simulink model "uas_sim"  (R2023a)
settings: Solver=VariableStepAuto  StartTime=0.0  StopTime=10.0  RelTol=1e-3  SampleTimeConstraint=STIndependent
values from neighbouring files (symbols this model uses):
  framePeriod_s = 1/frameRate_hz    (= 0.02)    [setup.m]
undefined symbols (not defined in the file or in its folder): Aircraft, datetime, datevec, Earth, Env, Fmu, InitCond, Telem, WGS84
libraries: aerolibconvert2 x8, simulink x8, aerolibadyn x3, aerolibasang x3, aerolibtransform2 x2, aerolibgravity2 x2, aerolibatmos2 x1, sharedutil x1, aerolibbdyn x1, shared6dof x1
(part 1 of 4)
settings Model: Creator=brian  LastModifiedBy=lagerprocessor
settings SolverCC: AlgebraicLoopSolver=TrustRegion
settings DataIOCC: SaveOutput=off  SignalLogging=off  DSMLogging=off  SaveTime=off  ReturnWorkspaceOutputsName=Data
settings DebuggingCC: UnconnectedInputMsg=warning  UnconnectedOutputMsg=warning  UnconnectedLineMsg=warning
settings ModelReferenceCC: EnableRefExpFcnMdlSchedulingChecks=on
settings RTWCC: DLArmComputeVersion=19.05

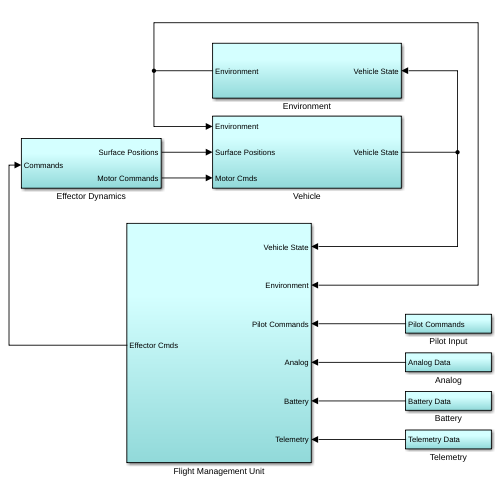
[thumbnail: Simulink's stored preview of the top-level diagram]
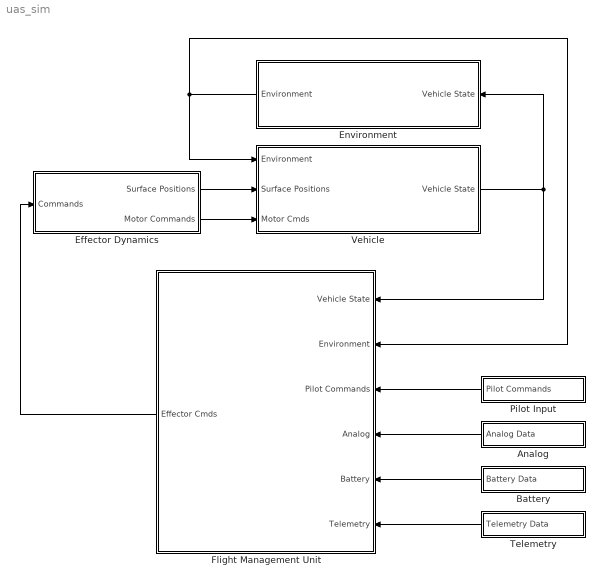
== system uas_sim ==
  Analog : Subsystem
  Battery : Subsystem
  Effector Dynamics : Subsystem
      settings: PortSchema="{\"entries\":[{\"content\":{\"sides\":[{\"content\":{\"connectorIds\":[]},\"type\":\"ConnectorPlacement.EquallySpacedRectSide\",\"uuid\":\"b20f7590-d69b-48b8-beb1-2fb7d3ab0357\"},{\"content\":{\"connectorIds\":[],\"side\":\"RIGHT\"},\"type\":\"ConnectorPlacement.EquallySpacedRectSide\",\"uuid\":\"07801f8a-7756-483e-a050-3c2fccc33404\"},{\"content\":{\"connectorIds\":[\"Out1\",\"Out2\"],\"side\":\"TOP\"},\"type\":\"ConnectorPlacement.EquallySpacedRectSide\",\"uuid\":\"ce3c3c94-ed36-4103-b079-69dcaeaf21e9\"},{\"content\":{\"connectorIds\":[\"In1\"],\"side\":\"BOTTOM\"},\"type\":\"ConnectorPlacement.EquallySpacedRectSide\",\"uuid\":\"ba78b819-a471-4bc3-b479-e6a973cfe14f\"},{\"content\":{\"connectorIds\":[],\"side\":\"HIDDEN\"},\"type\":\"ConnectorPlacement.EquallySpacedRectSide\",\"uuid\":\"3cf915a5-25a1-4380-9090-9561533312da\"}]},\"type\":\"ConnectorPlacement.EquallySpacedConnector\",\"uuid\":\"7ef4ddaa-ccd2-4778-89ce-8b4685524e82\"}],\"packageUris\":[\"http://schema.mathworks.com/mf0/Connector/R2020b\"],\"version\":\"1.0\"}"
  Environment : Subsystem
  Flight Management Unit : Subsystem
  Pilot Input : Subsystem
  Telemetry : Subsystem
  Vehicle : Subsystem
  wires:
  Vehicle/1(Vehicle State) -> Environment/1(Vehicle State), Flight Management Unit/1(Vehicle State)
  Pilot Input/1(Pilot Commands) -> Flight Management Unit/3(Pilot Commands)
  Environment/1(Environment) -> Vehicle/1(Environment), Flight Management Unit/2(Environment)
  Effector Dynamics/1(Surface Positions) -> Vehicle/2(Surface Positions)
  Effector Dynamics/2(Motor Commands) -> Vehicle/3(Motor Cmds)
  Telemetry/1(Telemetry Data) -> Flight Management Unit/6(Telemetry)
  Flight Management Unit/1(Effector Cmds) -> Effector Dynamics/1(Commands)
  Analog/1(Analog Data) -> Flight Management Unit/4(Analog)
  Battery/1(Battery Data) -> Flight Management Unit/5(Battery)

== system uas_sim/Analog ==
  note: Raw voltages measured at the FMU, should be between
      | 0 and 3.3V
  Bus Creator : BusCreator  Inputs=1
  Constant : Constant  Value=zeros(1, Fmu.NUM_AIN)
  Analog Data : Outport
  wires:
  Bus Creator/1 -> Analog Data/1
  Constant/1 -> Bus Creator/1  "Voltages"

== system uas_sim/Battery ==
  note: This is the amp draw from the battery
  note: The mRo Power Zero module
      | outputs 1V for 33.594 amps drawn
      | from the battery
  note: This is the voltage measured by the FMU
      | power port. It is typically the current, scaled
      | by the power module mA / volt
  note: This is the voltage
      | measured by the FMU at
      | the power port. It is typically
      | the battery voltage scaled by the
      | power module voltage divider.
  note: The mRo Power Zero module
      | outputs 1V for 15.30 V at the
      | battery
  Bus Creator : BusCreator  Inputs=2
  Constant : Constant  Value=Aircraft.Battery.voltage
  Constant1 : Constant  Value=42
  Constant2 : Constant  Value=33.594
  Constant3 : Constant  Value=15.30
  Divide : Product  Inputs=*/
  Divide1 : Product  Inputs=*/
  Battery Data : Outport
  wires:
  Bus Creator/1 -> Battery Data/1
  Constant2/1 -> Divide/2
  Constant1/1 -> Divide/1
  Divide/1 -> Bus Creator/2  "Current [V]"
  Divide1/1 -> Bus Creator/1  "Voltage [V]"
  Constant/1 -> Divide1/1
  Constant3/1 -> Divide1/2

== system uas_sim/Effector Dynamics ==
  Commands : Inport
  Actuator Dynamics : Subsystem
  Add : Sum
  Add1 : Sum
  Bus Selector : BusSelector  OutputSignals=PWM.Cmds,SBUS.Cmds
  Constant : Constant  Value=InitCond.surf_rad
  Constant1 : Constant  Value=InitCond.motor_cmd
  Mux : Mux  Inputs=2
  Selector : Selector  InputPortWidth=Aircraft.Eff.nCh  IndexOptions=Index vector (dialog)  Indices=Aircraft.Surf.map  OutputSizes=1
  Selector1 : Selector  InputPortWidth=Aircraft.Eff.nCh  IndexOptions=Index vector (dialog)  Indices=Aircraft.Motor.map  OutputSizes=1
  Surface Positions : Outport
  Motor Commands : Outport  Port=2
  wires:
  Commands/1 -> Bus Selector/1
  Bus Selector/1 -> Mux/1  "<Cmds>"
  Bus Selector/2 -> Mux/2  "<Cmds>"
  Mux/1 -> Selector1/1, Selector/1
  Actuator Dynamics/1(Position) -> Surface Positions/1
  Selector/1 -> Add/2
  Add/1 -> Actuator Dynamics/1(Command)
  Constant/1 -> Add/1
  Add1/1 -> Motor Commands/1
  Selector1/1 -> Add1/1
  Constant1/1 -> Add1/2

== system uas_sim/Environment ==
  note: nT to uT conversion
  Vehicle State : Inport
  Angle Conversion4 : aerolibconvert2/Angle Conversion  IU=rad  OU=deg
  Angle Conversion5 : aerolibconvert2/Angle Conversion  IU=rad  OU=deg
  Bus Creator : BusCreator  Inputs=6
  Bus Selector : BusSelector  OutputSignals=Latitude [rad],Longitude [rad],Altitude WGS84 [m],Altitude MSL [m]
  COESA Atmosphere Model : aerolibatmos2/COESA Atmosphere Model  units=Metric (MKS)  spec=1976 COESA-extended U.S. Standard Atmosphere  model=Profile  profile_var=High temperature  profile_percent=1%  profile_alt=5 km (16404 ft)  envelope_var=High temperature  envelope_percent=1%  action=Warning
  Constant : Constant  Value=Env.wmm_nt
  Gain : Gain  Gain=1e-3
  Mux : Mux  Inputs=3
  "WGS84 Gravity Model  " : GravityWGS84
  Environment : Outport
  wires:
  [lon_deg] -> Mux/2
  COESA Atmosphere Model/4 -> Bus Creator/4  "Density [kg/m^3]"
  Mux/1 -> "WGS84 Gravity Model  "/1
  Bus Selector/3 -> [alt_wgs84_m]  "<Altitude WGS84 [m]>"
  Vehicle State/1 -> Bus Selector/1
  Bus Selector/2 -> Angle Conversion5/1  "<Longitude [rad]>"
  COESA Atmosphere Model/2 -> Bus Creator/2  "Speed of Sound [m/s]"
  Bus Selector/4 -> COESA Atmosphere Model/1  "<Altitude MSL [m]>"
  [alt_wgs84_m] -> Mux/3
  Angle Conversion4/1 -> [lat_deg]
  [lat_deg] -> Mux/1
  Bus Creator/1 -> Environment/1
  Constant/1 -> Gain/1
  Gain/1 -> Bus Creator/6  "Magnetic Field [uT]"
  "WGS84 Gravity Model  "/1 -> Bus Creator/5  "Gravity [m/s/s]"
  Bus Selector/1 -> Angle Conversion4/1  "<Latitude [rad]>"
  COESA Atmosphere Model/3 -> Bus Creator/3  "Pressure [Pa]"
  COESA Atmosphere Model/1 -> Bus Creator/1  "Temperature [K]"
  Angle Conversion5/1 -> [lon_deg]

== system uas_sim/Flight Management Unit ==
  Vehicle State : Inport
  Environment : Inport  Port=2
  Pilot Commands : Inport  Port=3
  Analog : Inport  Port=4
  Battery : Inport  Port=5
  Telemetry : Inport  Port=6
  Bus Selector : BusSelector  OutputSignals=SBUS,PWM  OutputAsBus=on
  Navigation Filter Model : Subsystem
      settings: PortSchema="{\"entries\":[{\"content\":{\"sides\":[{\"content\":{\"connectorIds\":[]},\"type\":\"ConnectorPlacement.EquallySpacedRectSide\",\"uuid\":\"b20f7590-d69b-48b8-beb1-2fb7d3ab0357\"},{\"content\":{\"connectorIds\":[],\"side\":\"RIGHT\"},\"type\":\"ConnectorPlacement.EquallySpacedRectSide\",\"uuid\":\"07801f8a-7756-483e-a050-3c2fccc33404\"},{\"content\":{\"connectorIds\":[\"In1\",\"In2\"],\"side\":\"TOP\"},\"type\":\"ConnectorPlacement.EquallySpacedRectSide\",\"uuid\":\"ce3c3c94-ed36-4103-b079-69dcaeaf21e9\"},{\"content\":{\"connectorIds\":[\"Out1\"],\"side\":\"BOTTOM\"},\"type\":\"ConnectorPlacement.EquallySpacedRectSide\",\"uuid\":\"ba78b819-a471-4bc3-b479-e6a973cfe14f\"},{\"content\":{\"connectorIds\":[],\"side\":\"HIDDEN\"},\"type\":\"ConnectorPlacement.EquallySpacedRectSide\",\"uuid\":\"3cf915a5-25a1-4380-9090-9561533312da\"}]},\"type\":\"ConnectorPlacement.EquallySpacedConnector\",\"uuid\":\"7ef4ddaa-ccd2-4778-89ce-8b4685524e82\"}],\"packageUris\":[\"http://schema.mathworks.com/mf0/Connector/R2020b\"],\"version\":\"1.0\"}"
  Sensor Models : Subsystem
      settings: PortSchema="{\"entries\":[{\"content\":{\"sides\":[{\"content\":{\"connectorIds\":[]},\"type\":\"ConnectorPlacement.EquallySpacedRectSide\",\"uuid\":\"b20f7590-d69b-48b8-beb1-2fb7d3ab0357\"},{\"content\":{\"connectorIds\":[],\"side\":\"RIGHT\"},\"type\":\"ConnectorPlacement.EquallySpacedRectSide\",\"uuid\":\"07801f8a-7756-483e-a050-3c2fccc33404\"},{\"content\":{\"connectorIds\":[\"In1\",\"In2\",\"In3\",\"In4\",\"In5\"],\"side\":\"TOP\"},\"type\":\"ConnectorPlacement.EquallySpacedRectSide\",\"uuid\":\"ce3c3c94-ed36-4103-b079-69dcaeaf21e9\"},{\"content\":{\"connectorIds\":[\"Out1\"],\"side\":\"BOTTOM\"},\"type\":\"ConnectorPlacement.EquallySpacedRectSide\",\"uuid\":\"ba78b819-a471-4bc3-b479-e6a973cfe14f\"},{\"content\":{\"connectorIds\":[],\"side\":\"HIDDEN\"},\"type\":\"ConnectorPlacement.EquallySpacedRectSide\",\"uuid\":\"3cf915a5-25a1-4380-9090-9561533312da\"}]},\"type\":\"ConnectorPlacement.EquallySpacedConnector\",\"uuid\":\"7ef4ddaa-ccd2-4778-89ce-8b4685524e82\"}],\"packageUris\":[\"http://schema.mathworks.com/mf0/Connector/R2020b\"],\"version\":\"1.0\"}"
  System Model : Subsystem
      settings: PortSchema="{\"entries\":[{\"content\":{\"sides\":[{\"content\":{\"connectorIds\":[]},\"type\":\"ConnectorPlacement.EquallySpacedRectSide\",\"uuid\":\"b20f7590-d69b-48b8-beb1-2fb7d3ab0357\"},{\"content\":{\"connectorIds\":[],\"side\":\"RIGHT\"},\"type\":\"ConnectorPlacement.EquallySpacedRectSide\",\"uuid\":\"07801f8a-7756-483e-a050-3c2fccc33404\"},{\"content\":{\"connectorIds\":[],\"side\":\"TOP\"},\"type\":\"ConnectorPlacement.EquallySpacedRectSide\",\"uuid\":\"ce3c3c94-ed36-4103-b079-69dcaeaf21e9\"},{\"content\":{\"connectorIds\":[\"Out1\"],\"side\":\"BOTTOM\"},\"type\":\"ConnectorPlacement.EquallySpacedRectSide\",\"uuid\":\"ba78b819-a471-4bc3-b479-e6a973cfe14f\"},{\"content\":{\"connectorIds\":[],\"side\":\"HIDDEN\"},\"type\":\"ConnectorPlacement.EquallySpacedRectSide\",\"uuid\":\"3cf915a5-25a1-4380-9090-9561533312da\"}]},\"type\":\"ConnectorPlacement.EquallySpacedConnector\",\"uuid\":\"7ef4ddaa-ccd2-4778-89ce-8b4685524e82\"}],\"packageUris\":[\"http://schema.mathworks.com/mf0/Connector/R2020b\"],\"version\":\"1.0\"}"
  Unit Delay : UnitDelay  SampleTime=-1  HasFrameUpgradeWarning=on
  Unit Delay1 : UnitDelay  SampleTime=-1  HasFrameUpgradeWarning=on
  Vehicle Management System (VMS) : Subsystem  TreatAsAtomicUnit=on
  Effector Cmds : Outport
  wires:
  Environment/1 -> Navigation Filter Model/1(Environment), Sensor Models/1(Environment)
  Vehicle State/1 -> Navigation Filter Model/2(Vehicle State), Sensor Models/2(Vehicle State)
  Sensor Models/1(Sensors) -> Unit Delay/1
  Navigation Filter Model/1(Navigation Filter Data) -> Unit Delay1/1
  System Model/1(System) -> Vehicle Management System (VMS)/1(System Data)
  Pilot Commands/1 -> Sensor Models/3(Inceptor Data)
  Telemetry/1 -> Vehicle Management System (VMS)/4(Telemetry Data)
  Vehicle Management System (VMS)/1(VMS Data) -> Bus Selector/1
  Bus Selector/1 -> Effector Cmds/1
  Unit Delay/1 -> Vehicle Management System (VMS)/2(Sensor Data)
  Unit Delay1/1 -> Vehicle Management System (VMS)/3(Navigation Filter Data)
  Analog/1 -> Sensor Models/4(Analog Data)
  Battery/1 -> Sensor Models/5(Battery Data)

== system uas_sim/Pilot Input ==
  note: SBUS Data:
      | New data: whether new SBUS data was received
      | Lost Frame: whether a frame of data was lost from the transmitter to receiver
      | Failsafe: the receiver enters failsafe mode when many lost frames occur in a row
      | Ch 17 / Ch 18: two boolean (on / off) values availble on some SBUS transmitters and receivers
      | Channel Data: 16 channels of data from transmitter sticks and switches. 11 bits wide limiting values to 0 - 2048. Actual ranges may be different, for example, FrSky typically uses 172 - 1811 unless its range is extended to +/- 150%
  Bus Creator : BusCreator  Inputs=6
  Constant : Constant  Value=0  OutDataTypeStr=int8
  Constant1 : Constant  Value=zeros(1, 16)  OutDataTypeStr=int8
  Constant2 : Constant  OutDataTypeStr=boolean
  Constant3 : Constant  Value=0  OutDataTypeStr=boolean
  Constant8 : Constant  Value=0  OutDataTypeStr=boolean
  Constant9 : Constant  Value=0  OutDataTypeStr=boolean
  Pilot Commands : Outport
  wires:
  Bus Creator/1 -> Pilot Commands/1
  Constant2/1 -> Bus Creator/1  "New Data"
  Constant8/1 -> Bus Creator/2  "Lost Frame"
  Constant9/1 -> Bus Creator/3  "Failsafe"
  Constant3/1 -> Bus Creator/4  "Ch 17"
  Constant/1 -> Bus Creator/5  "Ch 18"
  Constant1/1 -> Bus Creator/6  "Channel Data"

== system uas_sim/Telemetry ==
  Bus Creator : BusCreator  Inputs=11
  Constant1 : Constant  Value=0  OutDataTypeStr=boolean
  Constant10 : Constant  Value=Telem.Fence  OutDataTypeStr=Bus: MissionItem
  Constant11 : Constant  Value=Telem.Rally  OutDataTypeStr=Bus: MissionItem
  Constant2 : Constant  Value=0  OutDataTypeStr=boolean
  Constant{3..6} (4 alike) : Constant  Value=0  OutDataTypeStr=int16
  Constant7 : Constant  Value=[0 0 0 0 0 0 0 0 0 0 0 0 0 0 0 0 0 0 0 0 0 0 0 0]  OutDataTypeStr=boolean
  Constant8 : Constant  Value=0  OutDataTypeStr=boolean
  Constant9 : Constant  Value=Telem.FlightPlan  OutDataTypeStr=Bus: MissionItem
  Telemetry Data : Outport
  wires:
  Bus Creator/1 -> Telemetry Data/1
  Constant8/1 -> Bus Creator/1  "Waypoints Updated"
  Constant1/1 -> Bus Creator/2  "Fence Updated"
  Constant2/1 -> Bus Creator/3  "Rally Points Updated"
  Constant3/1 -> Bus Creator/4  "Current Waypoint Index"
  Constant4/1 -> Bus Creator/5  "Number of Waypoints"
  Constant5/1 -> Bus Creator/6  "Number of Fence Points"
  Constant6/1 -> Bus Creator/7  "Number of Rally Points"
  Constant7/1 -> Bus Creator/8  "Parameters"
  Constant9/1 -> Bus Creator/9  "Flight Plan"
  Constant10/1 -> Bus Creator/10  "Fence"
  Constant11/1 -> Bus Creator/11  "Rally"

== system uas_sim/Vehicle ==
  Environment : Inport
  Surface Positions : Inport  Port=2  PortDimensions=Aircraft.Surf.nSurf
  Motor Cmds : Inport  Port=3
  Bus Creator : BusCreator  Inputs=26
  Bus Selector : BusSelector  OutputSignals=Gravity [m/s/s],Density [kg/m^3],Speed of Sound [m/s]
  Bus Selector1 : BusSelector  OutputSignals=Body Velocity [m/s],Body Rotational Rate [rad/s],Dynamic Pressure [Pa],Airspeed [m/s],Angle of Attack [rad],Sideslip Angle [rad],DCM_be
  Forces and Moments : Subsystem
  Vehicle Model : Subsystem
  Vehicle State : Outport
  wires:
  Bus Selector/1 -> Forces and Moments/10(Gravity [m/s/s])  "<Gravity [m/s/s]>"
  Bus Selector1/1 -> Forces and Moments/1(Body Velocity [m/s])  "<Body Velocity [m/s]>"
  Bus Selector1/2 -> Forces and Moments/2(Body Rotational Rate [rad/s])  "<Body Rotational Rate [rad/s]>"
  Vehicle Model/20(Angle of Attack Rate [rad/s]) -> Bus Creator/20  "Angle of Attack Rate [rad/s]"
  Bus Selector1/4 -> Forces and Moments/4(Airspeed [m/s])  "<Airspeed [m/s]>"
  Bus Selector1/6 -> Forces and Moments/6(Sideslip Angle [rad])  "<Sideslip Angle [rad]>"
  Bus Selector1/3 -> Forces and Moments/3(Dynamic Pressure [Pa])  "<Dynamic Pressure [Pa]>"
  Vehicle Model/4(Altitude MSL [m]) -> Bus Creator/4  "Altitude MSL [m]"
  Vehicle Model/26(DCM_be) -> Bus Creator/26  "DCM_be"
  Vehicle Model/16(Dynamic Pressure [Pa]) -> Bus Creator/16  "Dynamic Pressure [Pa]"
  Vehicle Model/22(Sideslip Angle Rate [rad/s]) -> Bus Creator/22  "Sideslip Angle Rate [rad/s]"
  Vehicle Model/21(Sideslip Angle [rad]) -> Bus Creator/21  "Sideslip Angle [rad]"
  Vehicle Model/24(Flight Path Angle [rad]) -> Bus Creator/24  "Flight Path Angle [rad]"
  Vehicle Model/11(Yaw [rad]) -> Bus Creator/11  "Yaw [rad]"
  Vehicle Model/18(Mach) -> Bus Creator/18  "Mach"
  Vehicle Model/5(Altitude AGL [m]) -> Bus Creator/5  "Altitude AGL [m]"
  Bus Selector1/7 -> Forces and Moments/7(DCM_be)  "<DCM_be>"
  Bus Selector1/5 -> Forces and Moments/5(Angle of Attack [rad])  "<Angle of Attack [rad]>"
  Bus Selector/2 -> Forces and Moments/11(Density [kg/m^3]), Vehicle Model/3(Density [kg/m^3])  "<Density [kg/m^3]>"
  Vehicle Model/6(NED Position [m]) -> Bus Creator/6  "NED Position [m]"
  Vehicle Model/23(Ground Track [rad]) -> Bus Creator/23  "Ground Track [rad]"
  Vehicle Model/10(Roll [rad]) -> Bus Creator/10  "Roll [rad]"
  Vehicle Model/7(NED Velocity [m/s]) -> Bus Creator/7  "NED Velocity [m/s]"
  Surface Positions/1 -> Forces and Moments/8(Surface Positions [rad])
  Vehicle Model/17(Airspeed [m/s]) -> Bus Creator/17  "Airspeed [m/s]"
  Vehicle Model/15(Body Rotational Accel [rad/s/s]) -> Bus Creator/15  "Body Rotational Accel [rad/s/s]"
  Vehicle Model/14(Body Rotational Rate [rad/s]) -> Bus Creator/14  "Body Rotational Rate [rad/s]"
  Vehicle Model/13(Body Accel [m/s/s]) -> Bus Creator/13  "Body Accel [m/s/s]"
  Vehicle Model/9(Pitch [rad]) -> Bus Creator/9  "Pitch [rad]"
  Vehicle Model/8(NED Accel [m/s/s]) -> Bus Creator/8  "NED Accel [m/s/s]"
  Forces and Moments/2(Mxyz [N-m]) -> Vehicle Model/2(Mxyz [N-m])
  Environment/1 -> Bus Selector/1
  Bus Selector/3 -> Vehicle Model/4(Speed of Sound [m/s])  "<Speed of Sound [m/s]>"
  Bus Creator/1 -> Bus Selector1/1, Vehicle State/1
  Forces and Moments/1(Fxyz [N]) -> Vehicle Model/1(Fxyz [N])
  Vehicle Model/19(Angle of Attack [rad]) -> Bus Creator/19  "Angle of Attack [rad]"
  Vehicle Model/3(Altitude WGS84 [m]) -> Bus Creator/3  "Altitude WGS84 [m]"
  Motor Cmds/1 -> Forces and Moments/9(Motor Cmds)
  Vehicle Model/2(Longitude [rad]) -> Bus Creator/2  "Longitude [rad]"
  Vehicle Model/1(Latitude [rad]) -> Bus Creator/1  "Latitude [rad]"
  Vehicle Model/12(Body Velocity [m/s]) -> Bus Creator/12  "Body Velocity [m/s]"
  Vehicle Model/25(Ground Speed [m/s]) -> Bus Creator/25  "Ground Speed [m/s]"

== system uas_sim/Effector Dynamics/Actuator Dynamics ==
  Command : Inport
  Integrator : Integrator  InitialCondition=InitCond.surf_rad  LimitOutput=on  UpperSaturationLimit=Aircraft.Surf.Limit.pos_deg  LowerSaturationLimit=Aircraft.Surf.Limit.neg_deg
  Saturation : Saturate  UpperLimit=Aircraft.Surf.Limit.rate_dps  LowerLimit=-Aircraft.Surf.Limit.rate_dps
  Sum : Sum  Inputs=-+|
  Position : Outport
  wires:
  Command/1 -> Sum/2
  Saturation/1 -> Integrator/1
  Integrator/1 -> Position/1, Sum/1
  Sum/1 -> Saturation/1

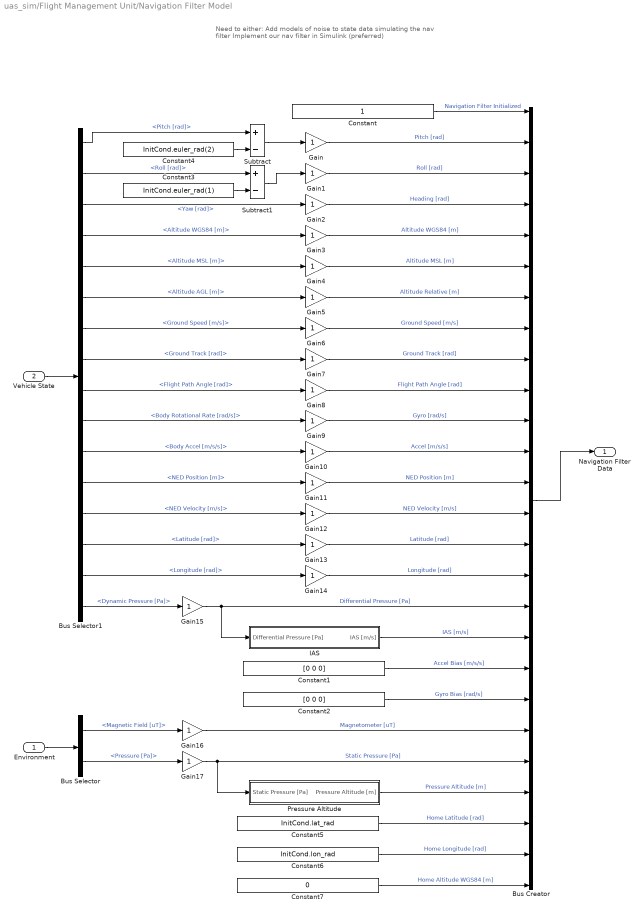
== system uas_sim/Flight Management Unit/Navigation Filter Model ==
  note: Need to either:
      | Add models of noise to state data simulating the nav filter
      | Implement our nav filter in Simulink (preferred)
  Environment : Inport
  Vehicle State : Inport  Port=2
  Bus Creator : BusCreator  Inputs=26
  Bus Selector : BusSelector  OutputSignals=Magnetic Field [uT],Pressure [Pa]
  Bus Selector1 : BusSelector  OutputSignals=Pitch [rad],Roll [rad],Yaw [rad],Altitude WGS84 [m],Altitude MSL [m],Altitude AGL [m],Ground Speed [m/s],Ground Track [rad],Flight Path Angle [rad],Body Rotational Rate [rad/s],Body Accel [m/s/s],NED Position [m],NED Velocity [m/s],Latitude [rad],Longitude [rad],Dynamic Pressure [Pa]
  Constant : Constant
  Constant1 : Constant  Value=[0 0 0]
  Constant2 : Constant  Value=[0 0 0]
  Constant3 : Constant  Value=InitCond.euler_rad(1)
  Constant4 : Constant  Value=InitCond.euler_rad(2)
  Constant5 : Constant  Value=InitCond.lat_rad
  Constant6 : Constant  Value=InitCond.lon_rad
  Constant7 : Constant  Value=0
  Gain{,1..17} (18 alike) : Gain
  IAS : Subsystem
  Pressure Altitude : Subsystem
  Subtract : Sum  Inputs=+-
  Subtract1 : Sum  Inputs=+-
  Navigation Filter Data : Outport
  wires:
  Environment/1 -> Bus Selector/1
  Bus Creator/1 -> Navigation Filter Data/1
  Vehicle State/1 -> Bus Selector1/1
  Constant/1 -> Bus Creator/1  "Navigation Filter Initialized"
  Bus Selector1/1 -> Subtract/1  "<Pitch [rad]>"
  Bus Selector1/2 -> Subtract1/1  "<Roll [rad]>"
  Bus Selector1/3 -> Gain2/1  "<Yaw [rad]>"
  Bus Selector1/4 -> Gain3/1  "<Altitude WGS84 [m]>"
  Bus Selector1/5 -> Gain4/1  "<Altitude MSL [m]>"
  Bus Selector1/6 -> Gain5/1  "<Altitude AGL [m]>"
  Bus Selector1/7 -> Gain6/1  "<Ground Speed [m/s]>"
  Bus Selector1/8 -> Gain7/1  "<Ground Track [rad]>"
  Bus Selector1/9 -> Gain8/1  "<Flight Path Angle [rad]>"
  Bus Selector1/10 -> Gain9/1  "<Body Rotational Rate [rad/s]>"
  Bus Selector1/11 -> Gain10/1  "<Body Accel [m/s/s]>"
  Bus Selector1/12 -> Gain11/1  "<NED Position [m]>"
  Bus Selector1/13 -> Gain12/1  "<NED Velocity [m/s]>"
  Bus Selector/2 -> Gain17/1  "<Pressure [Pa]>"
  Pressure Altitude/1(Pressure Altitude [m]) -> Bus Creator/23  "Pressure Altitude [m]"
  Bus Selector/1 -> Gain16/1  "<Magnetic Field [uT]>"
  Constant2/1 -> Bus Creator/20  "Gyro Bias [rad/s]"
  Constant1/1 -> Bus Creator/19  "Accel Bias [m/s/s]"
  IAS/1(IAS [m/s]) -> Bus Creator/18  "IAS [m/s]"
  Bus Selector1/16 -> Gain15/1  "<Dynamic Pressure [Pa]>"
  Bus Selector1/15 -> Gain14/1  "<Longitude [rad]>"
  Bus Selector1/14 -> Gain13/1  "<Latitude [rad]>"
  Gain/1 -> Bus Creator/2  "Pitch [rad]"
  Gain1/1 -> Bus Creator/3  "Roll [rad]"
  Gain2/1 -> Bus Creator/4  "Heading [rad]"
  Gain3/1 -> Bus Creator/5  "Altitude WGS84 [m]"
  Gain4/1 -> Bus Creator/6  "Altitude MSL [m]"
  Gain5/1 -> Bus Creator/7  "Altitude Relative [m]"
  Gain6/1 -> Bus Creator/8  "Ground Speed [m/s]"
  Gain7/1 -> Bus Creator/9  "Ground Track [rad]"
  Gain8/1 -> Bus Creator/10  "Flight Path Angle [rad]"
  Gain9/1 -> Bus Creator/11  "Gyro [rad/s]"
  Gain10/1 -> Bus Creator/12  "Accel [m/s/s]"
  Gain11/1 -> Bus Creator/13  "NED Position [m]"
  Gain12/1 -> Bus Creator/14  "NED Velocity [m/s]"
  Gain13/1 -> Bus Creator/15  "Latitude [rad]"
  Gain14/1 -> Bus Creator/16  "Longitude [rad]"
  Gain15/1 -> IAS/1(Differential Pressure [Pa]), Bus Creator/17  "Differential Pressure [Pa]"
  Gain16/1 -> Bus Creator/21  "Magnetometer [uT]"
  Gain17/1 -> Pressure Altitude/1(Static Pressure [Pa]), Bus Creator/22  "Static Pressure [Pa]"
  Subtract/1 -> Gain/1
  Subtract1/1 -> Gain1/1
  Constant3/1 -> Subtract1/2
  Constant4/1 -> Subtract/2
  Constant5/1 -> Bus Creator/24  "Home Latitude [rad]"
  Constant6/1 -> Bus Creator/25  "Home Longitude [rad]"
  Constant7/1 -> Bus Creator/26  "Home Altitude WGS84 [m]"

== system uas_sim/Flight Management Unit/Sensor Models ==
  Environment : Inport
  Vehicle State : Inport  Port=2
  Inceptor Data : Inport  Port=3
  Analog Data : Inport  Port=4
  Battery Data : Inport  Port=5
  Bus Creator : BusCreator  Inputs=8
  Bus Selector : BusSelector  OutputSignals=Body Rotational Rate [rad/s],Body Accel [m/s/s],DCM_be
  Bus Selector1 : BusSelector  OutputSignals=Latitude [rad],Longitude [rad],Altitude WGS84 [m],NED Velocity [m/s]
  Bus Selector2 : BusSelector  OutputSignals=Dynamic Pressure [Pa]
  Bus Selector3 : BusSelector  OutputSignals=Gravity [m/s/s],Magnetic Field [uT]
  Bus Selector4 : BusSelector  OutputSignals=Pressure [Pa]
  Constant : Constant  Value=Aircraft.Sensors.PitotStaticInstalled
  Diff Pressure Sensor : Subsystem
  GNSS : Subsystem
  IMU : Subsystem
  Static Pressure Sensor : Subsystem
  Sensors : Outport
  wires:
  Bus Creator/1 -> Sensors/1
  Vehicle State/1 -> Bus Selector2/1, Bus Selector1/1, Bus Selector/1
  Bus Selector/1 -> IMU/1(Body Rotational Rate [rad/s])  "<Body Rotational Rate [rad/s]>"
  Bus Selector/2 -> IMU/2(Body Accel [m/s/s])  "<Body Accel [m/s/s]>"
  Bus Selector/3 -> IMU/3(DCM_be)  "<DCM_be>"
  Bus Selector1/1 -> GNSS/1(Latitude [rad])  "<Latitude [rad]>"
  Bus Selector1/2 -> GNSS/2("Longitude [rad] ")  "<Longitude [rad]>"
  Bus Selector1/3 -> GNSS/3(Altitude WGS84 [m])  "<Altitude WGS84 [m]>"
  Bus Selector1/4 -> GNSS/4(NED Velocity [m/s])  "<NED Velocity [m/s]>"
  Bus Selector2/1 -> Diff Pressure Sensor/1(Pressure)  "<Dynamic Pressure [Pa]>"
  Environment/1 -> Bus Selector4/1, Bus Selector3/1
  Bus Selector3/1 -> IMU/4(Gravity [m/s/s])  "<Gravity [m/s/s]>"
  Bus Selector3/2 -> IMU/5(Magnetic Field [uT])  "<Magnetic Field [uT]>"
  Bus Selector4/1 -> Static Pressure Sensor/1(Pressure)  "<Pressure [Pa]>"
  IMU/1(IMU Data) -> Bus Creator/4  "IMU"
  GNSS/1(GNSS Data) -> Bus Creator/5  "GNSS"
  Inceptor Data/1 -> Bus Creator/2  "Inceptor"
  Diff Pressure Sensor/1(Pressure Data) -> Bus Creator/7  "Differential Pressure"
  Static Pressure Sensor/1(Pressure Data) -> Bus Creator/6  "Static Pressure"
  Constant/1 -> Bus Creator/1  "Pitot Static Installed"
  Analog Data/1 -> Bus Creator/3  "Analog"
  Battery Data/1 -> Bus Creator/8  "Battery"

== system uas_sim/Flight Management Unit/System Model ==
  Bus Creator : BusCreator  Inputs=6
  Clock : Clock
      settings: Decimation=1e6
  Constant : Constant  Value=5
  Constant1 : Constant  Value=5
  Constant2 : Constant  Value=5
  Constant3 : Constant  Value=Aircraft.Battery.voltage
  Constant4 : Constant  Value=framePeriod_s
  Gain : Gain  Gain=1e6
  Gain1 : Gain  Gain=1e6
  System : Outport
  wires:
  Clock/1 -> Gain/1  "System Time [s]"
  Bus Creator/1 -> System/1
  Constant4/1 -> Gain1/1  "Frame Time [s]"
  Gain1/1 -> Bus Creator/1  "Frame Time [us]"
  Constant3/1 -> Bus Creator/2  "Input Voltage"
  Constant2/1 -> Bus Creator/3  "Regulated Voltage"
  Constant1/1 -> Bus Creator/4  "PWM Voltage"
  Constant/1 -> Bus Creator/5  "SBUS Voltage"
  Gain/1 -> Bus Creator/6  "System Time [us]"

== system uas_sim/Flight Management Unit/Vehicle Management System (VMS) ==
  System Data : Inport
  Sensor Data : Inport  Port=2
  Navigation Filter Data : Inport  Port=3
  Telemetry Data : Inport  Port=4
  Variant Subsystem : Subsystem  Variant=on
  VMS Data : Outport
  wires:
  Variant Subsystem/1(VMS Data) -> VMS Data/1
  System Data/1 -> Variant Subsystem/1(System Data)
  Sensor Data/1 -> Variant Subsystem/2(Sensor Data)
  Navigation Filter Data/1 -> Variant Subsystem/3(Navigation Filter Data)
  Telemetry Data/1 -> Variant Subsystem/4(Telemetry Data)

== system uas_sim/Vehicle/Forces and Moments ==
  Body Velocity [m/s] : Inport
  Body Rotational Rate [rad/s] : Inport  Port=2
  Dynamic Pressure [Pa] : Inport  Port=3
  Airspeed [m/s] : Inport  Port=4
  Angle of Attack [rad] : Inport  Port=5
  Sideslip Angle [rad] : Inport  Port=6
  DCM_be : Inport  Port=7
  Surface Positions [rad] : Inport  Port=8
  Motor Cmds : Inport  Port=9
  Gravity [m/s/s] : Inport  Port=10
  Density [kg/m^3] : Inport  Port=11
  Add : Sum  Inputs=+++
  Aerodynamic : Subsystem
  Demux3 : Demux  Outputs=2
  Gravitational : Subsystem
  Propulsive : Subsystem
  Fxyz [N] : Outport
  Mxyz [N-m] : Outport  Port=2
  wires:
  Surface Positions [rad]/1 -> Aerodynamic/3(Surface Positions [rad])
  Add/1 -> Demux3/1
  Gravity [m/s/s]/1 -> Gravitational/1(Gravity [m/s/s])
  Motor Cmds/1 -> Propulsive/3(Motor Cmds)
  Demux3/1 -> Fxyz [N]/1
  Sideslip Angle [rad]/1 -> Aerodynamic/6(Sideslip Angle [rad])
  Dynamic Pressure [Pa]/1 -> Aerodynamic/4(Dynamic Pressure [Pa])
  DCM_be/1 -> Gravitational/2(DCM_be)
  Angle of Attack [rad]/1 -> Aerodynamic/5(Angle of Attack [rad])
  Propulsive/1(Fxyz Mxyz) -> Add/3
  Body Rotational Rate [rad/s]/1 -> Propulsive/2(Rotational Rate [rad/s]), Aerodynamic/2(Body Rotational Rates [rad/s])
  Demux3/2 -> Mxyz [N-m]/1
  Airspeed [m/s]/1 -> Propulsive/1(Airspeed [m/s]), Aerodynamic/7(Airspeed [m/s])
  Aerodynamic/1(Fxyz Mxzy) -> Add/1
  Body Velocity [m/s]/1 -> Aerodynamic/1(Body Velocity [m/s])
  Gravitational/1(Fxyz Mxyz) -> Add/2
  Density [kg/m^3]/1 -> Propulsive/4(Air Density [kg/m^3])

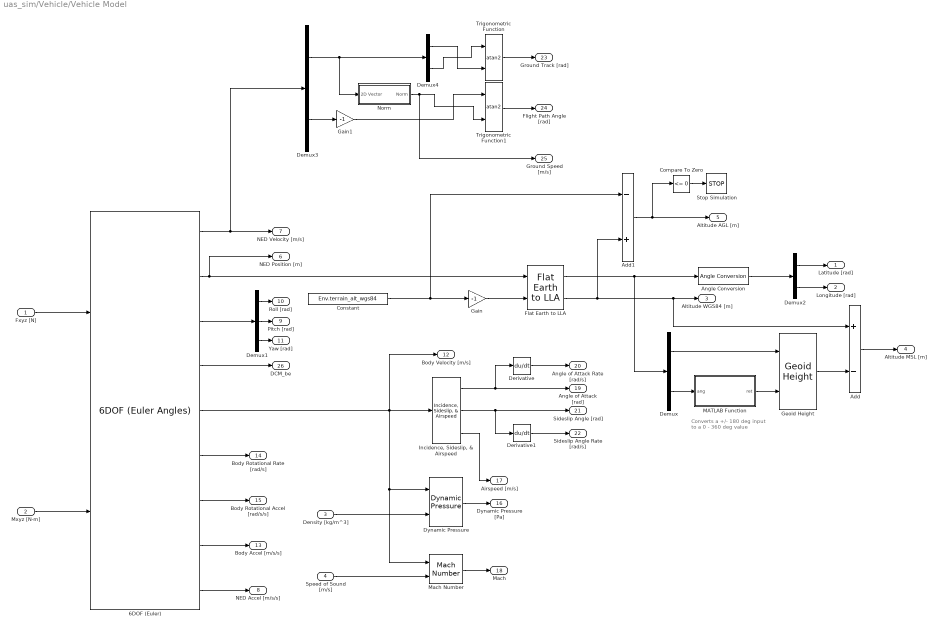
== system uas_sim/Vehicle/Vehicle Model ==
  note: Converts a +/- 180 deg
      | input to a 0 - 360 deg value
  Fxyz [N] : Inport
  Mxyz [N-m] : Inport  Port=2
  Density [kg/m^3] : Inport  Port=3
  Speed of Sound [m/s] : Inport  Port=4
  6DOF (Euler) : shared6dof/6DOF (Euler Angles)  units=Metric (MKS)  mtype=Fixed  rep=Euler Angles  xme_0=InitCond.ned_pos_m  Vm_0=InitCond.body_vel_mps  eul_0=InitCond.euler_rad  pm_0=InitCond.body_rot_rate_radps  mass_0=Aircraft.Mass.mass_kg  mass_e=0.5  mass_f=2.0  inertia=Aircraft.Mass.inertia_kgm2  inertia_e=eye(3)  inertia_f=2*eye(3)  k_quat=1.0  vre_flag=on  abi_flag=on  aMode=0  xme_statename=''  Vm_statename=''  eul_statename=''  quat_statename=''  pm_statename=''  mass_statename=''
  Add : Sum  Inputs=+-
  Add1 : Sum  Inputs=-+
  Angle Conversion : aerolibconvert2/Angle Conversion  IU=deg  OU=rad
  Compare To Zero : simulink/Logic and Bit Operations/Compare To Zero  relop=<=  OutDataTypeStr=boolean
  Constant : Constant  Value=Env.terrain_alt_wgs84
  Demux : Demux  Outputs=2
  Demux1 : Demux  Outputs=3
  Demux2 : Demux  Outputs=2
  Demux3 : Demux  Outputs=[2 1]
  Demux4 : Demux  Outputs=2
  Derivative : Derivative
  Derivative1 : Derivative
  Dynamic Pressure : aerolibasang/Dynamic Pressure
  Flat Earth to LLA : aerolibtransform2/Flat Earth to LLA  units=Metric (MKS)  ptype=Earth (WGS84)  F=1/298.257223563  R=6378137  refPosPort=off  LL0=[rad2deg(InitCond.lat_rad) rad2deg(InitCond.lon_rad)]  psi=0
  Gain : Gain  Gain=-1
  Gain1 : Gain  Gain=-1
  Geoid Height : aerolibgravity2/Geoid Height  units=Metric (MKS)  gtype=EGM2008  datafile='geoidegm96grid'  dtype=double  action=Warning
  "Incidence, Sideslip, & Airspeed" : aerolibasang/Incidence, Sideslip, & Airspeed
  MATLAB Function : MATLAB Function  TreatAsAtomicUnit=on
  Mach Number : aerolibasang/Mach Number
  Norm : Subsystem
  Stop Simulation : Stop
  Trigonometric Function : Trigonometry  Operator=atan2
  Trigonometric Function1 : Trigonometry  Operator=atan2
  Latitude [rad] : Outport
  Longitude [rad] : Outport  Port=2
  Altitude WGS84 [m] : Outport  Port=3
  Altitude MSL [m] : Outport  Port=4
  Altitude AGL [m] : Outport  Port=5
  NED Position [m] : Outport  Port=6
  NED Velocity [m/s] : Outport  Port=7
  NED Accel [m/s/s] : Outport  Port=8
  Pitch [rad] : Outport  Port=9
  Roll [rad] : Outport  Port=10
  Yaw [rad] : Outport  Port=11
  Body Velocity [m/s] : Outport  Port=12
  Body Accel [m/s/s] : Outport  Port=13
  Body Rotational Rate [rad/s] : Outport  Port=14
  Body Rotational Accel [rad/s/s] : Outport  Port=15
  Dynamic Pressure [Pa] : Outport  Port=16
  Airspeed [m/s] : Outport  Port=17
  Mach : Outport  Port=18
  Angle of Attack [rad] : Outport  Port=19
  Angle of Attack Rate [rad/s] : Outport  Port=20
  Sideslip Angle [rad] : Outport  Port=21
  Sideslip Angle Rate [rad/s] : Outport  Port=22
  Ground Track [rad] : Outport  Port=23
  Flight Path Angle [rad] : Outport  Port=24
  Ground Speed [m/s] : Outport  Port=25
  DCM_be : Outport  Port=26
  wires:
  Fxyz [N]/1 -> 6DOF (Euler)/1
  Mxyz [N-m]/1 -> 6DOF (Euler)/2
  6DOF (Euler)/5 -> Body Velocity [m/s]/1, "Incidence, Sideslip, & Airspeed"/1, Dynamic Pressure/1, Mach Number/1
  Flat Earth to LLA/1 -> Demux/1, Angle Conversion/1
  Flat Earth to LLA/2 -> Add1/2, Add/1, Altitude WGS84 [m]/1
  Geoid Height/1 -> Add/2
  Demux/2 -> MATLAB Function/1(ang)
  Demux/1 -> Geoid Height/1
  "Incidence, Sideslip, & Airspeed"/3 -> Airspeed [m/s]/1
  Density [kg/m^3]/1 -> Dynamic Pressure/2
  Angle Conversion/1 -> Demux2/1
  6DOF (Euler)/4 -> DCM_be/1
  Demux1/1 -> Roll [rad]/1
  6DOF (Euler)/3 -> Demux1/1
  Demux1/2 -> Pitch [rad]/1
  Demux1/3 -> Yaw [rad]/1
  Dynamic Pressure/1 -> Dynamic Pressure [Pa]/1
  "Incidence, Sideslip, & Airspeed"/1 -> Derivative/1, Angle of Attack [rad]/1
  "Incidence, Sideslip, & Airspeed"/2 -> Derivative1/1, Sideslip Angle [rad]/1
  Add/1 -> Altitude MSL [m]/1
  Gain/1 -> Flat Earth to LLA/2
  Demux2/2 -> Longitude [rad]/1
  Demux2/1 -> Latitude [rad]/1
  6DOF (Euler)/2 -> NED Position [m]/1, Flat Earth to LLA/1
  6DOF (Euler)/6 -> Body Rotational Rate [rad/s]/1
  6DOF (Euler)/7 -> Body Rotational Accel [rad/s/s]/1
  6DOF (Euler)/8 -> Body Accel [m/s/s]/1
  6DOF (Euler)/1 -> Demux3/1, NED Velocity [m/s]/1
  MATLAB Function/1(ret) -> Geoid Height/2
  Demux3/1 -> Norm/1(2D Vector), Demux4/1
  Trigonometric Function/1 -> Ground Track [rad]/1
  Demux3/2 -> Gain1/1
  Gain1/1 -> Trigonometric Function1/1
  Norm/1(Norm) -> Ground Speed [m/s]/1, Trigonometric Function1/2
  Trigonometric Function1/1 -> Flight Path Angle [rad]/1
  6DOF (Euler)/9 -> NED Accel [m/s/s]/1
  Speed of Sound [m/s]/1 -> Mach Number/2
  Mach Number/1 -> Mach/1
  Derivative/1 -> Angle of Attack Rate [rad/s]/1
  Derivative1/1 -> Sideslip Angle Rate [rad/s]/1
  Constant/1 -> Add1/1, Gain/1
  Add1/1 -> Compare To Zero/1, Altitude AGL [m]/1
  Compare To Zero/1 -> Stop Simulation/1
  Demux4/1 -> Trigonometric Function/2
  Demux4/2 -> Trigonometric Function/1

== system uas_sim/Flight Management Unit/Navigation Filter Model/IAS ==
  note: Avoid negative values
  Differential Pressure [Pa] : Inport
  Add : Sum
  Constant : Constant  OutDataTypeStr=double
  Constant1 : Constant  Value=2/7  OutDataTypeStr=double
  Constant2 : Constant  OutDataTypeStr=double
  Divide : Product  Inputs=*/
  Multiply : Gain  Gain=5
  Pow : Math  Operator=pow  RndMeth=Zero
  Product : Product
  Saturation : Saturate  UpperLimit=inf  LowerLimit=0
  Sqrt : Sqrt
  Standard Sea Level Pressure [Pa] : Constant  Value=101325  OutDataTypeStr=double
  Standard Sea Level Speed of Sound [m/s] : Constant  Value=340.29  OutDataTypeStr=double
  Subtract : Sum  Inputs=+-
  IAS [m/s] : Outport
  wires:
  Differential Pressure [Pa]/1 -> Saturation/1
  Saturation/1 -> Divide/1
  Standard Sea Level Pressure [Pa]/1 -> Divide/2
  Divide/1 -> Add/1
  Constant/1 -> Add/2
  Constant1/1 -> Pow/2
  Add/1 -> Pow/1
  Pow/1 -> Subtract/1
  Constant2/1 -> Subtract/2
  Subtract/1 -> Multiply/1
  Multiply/1 -> Sqrt/1
  Sqrt/1 -> Product/1
  Product/1 -> IAS [m/s]/1
  Standard Sea Level Speed of Sound [m/s]/1 -> Product/2

== system uas_sim/Flight Management Unit/Navigation Filter Model/Pressure Altitude ==
  note: Avoid negative values
  Static Pressure [Pa] : Inport
  Acceleration due to Gravity [m/s/s] : Constant  Value=9.80665  OutDataTypeStr=double
  Constant : Constant  OutDataTypeStr=double
  Divide : Product  Inputs=*/
  Divide1 : Product  Inputs=*/
  Divide2 : Product  Inputs=*/*
  Gas Constant [J/kg/mol] : Constant  Value=8.31446261815324  OutDataTypeStr=double
  Lapse Rate [K/m] : Constant  Value=0.0065  OutDataTypeStr=double
  Lapse Rate [K/m]1 : Constant  Value=0.0065  OutDataTypeStr=double
  Molecular Mass Air [kg/mol] : Constant  Value=0.0289644  OutDataTypeStr=double
  Pow : Math  Operator=pow  RndMeth=Zero
  Product : Product
  Product1 : Product
  Saturation1 : Saturate  UpperLimit=inf  LowerLimit=0
  Standard Sea Level Pressure [Pa] : Constant  Value=101325  OutDataTypeStr=double
  Standard Sea Level Temperature [K] : Constant  Value=288.15  OutDataTypeStr=double
  Subtract : Sum  Inputs=+-
  Pressure Altitude [m] : Outport
  wires:
  Static Pressure [Pa]/1 -> Saturation1/1
  Saturation1/1 -> Divide/1
  Standard Sea Level Pressure [Pa]/1 -> Divide/2
  Divide/1 -> Pow/1
  Product1/1 -> Divide1/1
  Product/1 -> Divide1/2
  Molecular Mass Air [kg/mol]/1 -> Product/1
  Acceleration due to Gravity [m/s/s]/1 -> Product/2
  Gas Constant [J/kg/mol]/1 -> Product1/2
  Lapse Rate [K/m]/1 -> Product1/1
  Divide1/1 -> Pow/2
  Pow/1 -> Subtract/2
  Constant/1 -> Subtract/1
  Subtract/1 -> Divide2/3
  Divide2/1 -> Pressure Altitude [m]/1
  Lapse Rate [K/m]1/1 -> Divide2/2
  Standard Sea Level Temperature [K]/1 -> Divide2/1

== system uas_sim/Flight Management Unit/Sensor Models/Diff Pressure Sensor ==
  Pressure : Inport
  Add : Sum  Inputs=+++
  Band-Limited White Noise : simulink/Sources/Band-Limited White Noise  Cov=Aircraft.Sensors.DiffPres.noise_pa  Ts=0.1  seed=[23341]
  Bus Creator : BusCreator  Inputs=4
  Bus Creator1 : BusCreator  Inputs=4
  Constant : Constant  Value=Aircraft.Sensors.DiffPres.bias_pa
  Constant1 : Constant  Value=Aircraft.Sensors.DiffPres.scale_factor
  Constant2 : Constant  Value=23
  Constant3 : Constant
  Constant4 : Constant
  Constant{5..8} (4 alike) : Constant  Value=0
  Constant9 : Constant  Value=Aircraft.Sensors.PitotStaticInstalled
  Product : Product
  Saturation : Saturate  UpperLimit=Aircraft.Sensors.DiffPres.upper_limit_pa  LowerLimit=Aircraft.Sensors.DiffPres.lower_limit_pa
  Switch : Switch  Criteria=u2 > Threshold  SaturateOnIntegerOverflow=off  InputSameDT=off
  Pressure Data : Outport
  wires:
  Switch/1 -> Pressure Data/1
  Constant9/1 -> Switch/2
  Bus Creator/1 -> Switch/1
  Bus Creator1/1 -> Switch/3
  Constant7/1 -> Bus Creator1/1  "New Data"
  Constant6/1 -> Bus Creator1/2  "Healthy"
  Constant5/1 -> Bus Creator1/4  "Die Temperature [C]"
  Constant8/1 -> Bus Creator1/3  "Pressure [Pa]"
  Constant1/1 -> Product/2
  Pressure/1 -> Product/1
  Product/1 -> Add/3
  Add/1 -> Saturation/1
  Constant/1 -> Add/2
  Band-Limited White Noise/1 -> Add/1
  Saturation/1 -> Bus Creator/3  "Pressure [Pa]"
  Constant2/1 -> Bus Creator/4  "Die Temperature [C]"
  Constant3/1 -> Bus Creator/2  "Healthy"
  Constant4/1 -> Bus Creator/1  "New Data"

== system uas_sim/Flight Management Unit/Sensor Models/GNSS ==
  note: Simulates the lower sampling rate of GNSS receivers
  Latitude [rad] : Inport
  "Longitude [rad] " : Inport  Port=2
  Altitude WGS84 [m] : Inport  Port=3
  NED Velocity [m/s] : Inport  Port=4
  Band-Limited White Noise : simulink/Sources/Band-Limited White Noise  Cov=[Aircraft.Sensors.Gnss.horz_accuracy_m Aircraft.Sensors.Gnss.horz_accuracy_m Aircraft.Sensors.Gnss.vert_accuracy_m]  Ts=0.1  seed=[23341]
  Band-Limited White Noise2 : simulink/Sources/Band-Limited White Noise  Cov=Aircraft.Sensors.Gnss.vel_accuracy_mps * ones(3, 1)  Ts=0.1  seed=[23341]
  Bus Creator : BusCreator  Inputs=19
  Clock : Clock
  Pulse Generator : DiscretePulseGenerator  PulseType=Time based  Period=1/Aircraft.Sensors.Gnss.sample_rate_hz  PulseWidth=5
  Triggered Subsystem : Subsystem  TreatAsAtomicUnit=on
  GNSS Data : Outport
  wires:
  Bus Creator/1 -> GNSS Data/1
  NED Velocity [m/s]/1 -> Triggered Subsystem/4(NED Velocity [m/s])
  Altitude WGS84 [m]/1 -> Triggered Subsystem/3(Altitude WGS84 [m])
  "Longitude [rad] "/1 -> Triggered Subsystem/2("Longitude [rad] ")
  Clock/1 -> Triggered Subsystem/7(clock)
  Band-Limited White Noise/1 -> Triggered Subsystem/5(Position Noise [m])
  Pulse Generator/1 -> Triggered Subsystem/Trigger
  Band-Limited White Noise2/1 -> Triggered Subsystem/6(Velocity Noise [m/s])
  Latitude [rad]/1 -> Triggered Subsystem/1(Latitude [rad])
  Triggered Subsystem/1(New Data) -> Bus Creator/1  "New Data"
  Triggered Subsystem/2(Healthy) -> Bus Creator/2  "Healthy"
  Triggered Subsystem/3(Fix) -> Bus Creator/3  "Fix"
  Triggered Subsystem/4(Num Satellites) -> Bus Creator/4  "Num Satellites"
  Triggered Subsystem/5(Week) -> Bus Creator/5  "Week"
  Triggered Subsystem/6(TOW [ms]) -> Bus Creator/6  "TOW [ms]"
  Triggered Subsystem/7(Alt WGS84 [m]) -> Bus Creator/7  "Altitude WGS84 [m]"
  Triggered Subsystem/8(Alt MSL [m]) -> Bus Creator/8  "Altitude MSL [m]"
  Triggered Subsystem/9(HDOP) -> Bus Creator/9  "HDOP"
  Triggered Subsystem/10(VDOP) -> Bus Creator/10  "VDOP"
  Triggered Subsystem/11(Track [rad]) -> Bus Creator/11  "Track [rad]"
  Triggered Subsystem/12(Speed [m/s]) -> Bus Creator/12  "Speed [m/s]"
  Triggered Subsystem/13(Horizontal Accuracy [m]) -> Bus Creator/13  "Horizontal Accuracy [m]"
  Triggered Subsystem/14(Vertical Accuracy [m]) -> Bus Creator/14  "Vertical Accuracy [m]"
  Triggered Subsystem/15(Velocity Accuracy [m/s]) -> Bus Creator/15  "Velocity Accuracy [m/s]"
  Triggered Subsystem/16(Track Accuracy [rad]) -> Bus Creator/16  "Track Accuracy [rad]"
  Triggered Subsystem/17(NED Vel [m/s]) -> Bus Creator/17  "NED Velocity [m/s]"
  Triggered Subsystem/18(Lat [rad]) -> Bus Creator/18  "Latitude [rad]"
  Triggered Subsystem/19(Lon [rad]) -> Bus Creator/19  "Longitude [rad]"

== system uas_sim/Flight Management Unit/Sensor Models/IMU ==
  Body Rotational Rate [rad/s] : Inport
  Body Accel [m/s/s] : Inport  Port=2
  DCM_be : Inport  Port=3
  Gravity [m/s/s] : Inport  Port=4
  Magnetic Field [uT] : Inport  Port=5
  Accelerometer : Subsystem
  Bus Creator : BusCreator  Inputs=8
  Constant{,1..3} (4 alike) : Constant
  Constant4 : Constant  Value=23
  Gyro : Subsystem
  Magnetometer : Subsystem
  Product1 : Product  Multiplication=Matrix(*)
  Product2 : Product  Multiplication=Matrix(*)
  Reshape : Reshape  OutputDimensionality=Column vector (2-D)
  Reshape1 : Reshape
  Reshape2 : Reshape
  Reshape3 : Reshape  OutputDimensionality=Column vector (2-D)
  IMU Data : Outport
  wires:
  Body Accel [m/s/s]/1 -> Accelerometer/1(Body Accel [m/s/s]), Gyro/2(Body Accel [m/s/s])
  DCM_be/1 -> Product2/1, Product1/1
  Gravity [m/s/s]/1 -> Reshape/1
  Bus Creator/1 -> IMU Data/1
  Product2/1 -> Reshape1/1
  Reshape1/1 -> Accelerometer/2(Gravitational Accel in Body Frame [m/s/s])
  Body Rotational Rate [rad/s]/1 -> Gyro/1(Body Rotational Rate [rad/s])
  Reshape2/1 -> Magnetometer/1(Body Magnetic Field [uT])
  Product1/1 -> Reshape2/1
  Reshape3/1 -> Product1/2
  Magnetic Field [uT]/1 -> Reshape3/1
  Magnetometer/1(Magnetometer [uT]) -> Bus Creator/8  "Magnetometer [uT]"
  Accelerometer/1(Accelerometer [m/s/s]) -> Bus Creator/7  "Accelerometer [m/s/s]"
  Gyro/1(Gyro [rad/s]) -> Bus Creator/6  "Gyro [rad/s]"
  Reshape/1 -> Product2/2
  Constant1/1 -> Bus Creator/2  "New Magnetometer Data"
  Constant/1 -> Bus Creator/1  "New IMU Data"
  Constant2/1 -> Bus Creator/3  "IMU Healthy"
  Constant3/1 -> Bus Creator/4  "Magnetometer Healthy"
  Constant4/1 -> Bus Creator/5  "Die Temperature [C]"

== system uas_sim/Flight Management Unit/Sensor Models/Static Pressure Sensor ==
  Pressure : Inport
  Add : Sum  Inputs=+++
  Band-Limited White Noise : simulink/Sources/Band-Limited White Noise  Cov=Aircraft.Sensors.StaticPres.noise_pa  Ts=0.1  seed=[23341]
  Bus Creator : BusCreator  Inputs=4
  Constant : Constant  Value=Aircraft.Sensors.StaticPres.bias_pa
  Constant1 : Constant  Value=Aircraft.Sensors.StaticPres.scale_factor
  Constant2 : Constant  Value=23
  Constant3 : Constant
  Constant4 : Constant
  Product : Product
  Saturation : Saturate  UpperLimit=Aircraft.Sensors.StaticPres.upper_limit_pa  LowerLimit=Aircraft.Sensors.StaticPres.lower_limit_pa
  Pressure Data : Outport
  wires:
  Constant4/1 -> Bus Creator/1  "New Data"
  Constant3/1 -> Bus Creator/2  "Healthy"
  Constant2/1 -> Bus Creator/4  "Die Temperature [C]"
  Saturation/1 -> Bus Creator/3  "Pressure [Pa]"
  Band-Limited White Noise/1 -> Add/1
  Constant/1 -> Add/2
  Add/1 -> Saturation/1
  Product/1 -> Add/3
  Pressure/1 -> Product/1
  Constant1/1 -> Product/2
  Bus Creator/1 -> Pressure Data/1

== system uas_sim/Flight Management Unit/Vehicle Management System (VMS)/Variant Subsystem ==
  System Data : Inport
  Sensor Data : Inport  Port=2
  Navigation Filter Data : Inport  Port=3
  Telemetry Data : Inport  Port=4
  FMU v1 : Subsystem  VariantControl=Fmu.version == 1
  FMU v2 : Subsystem  VariantControl=Fmu.version == 3
  FMU v2 Beta : Subsystem  VariantControl=Fmu.version == 2
  VMS Data : Outport

== system uas_sim/Vehicle/Forces and Moments/Aerodynamic ==
  note: C6 = [CD, CY, CLift, CL, CM, CN]
  Body Velocity [m/s] : Inport
  Body Rotational Rates [rad/s] : Inport  Port=2
  Surface Positions [rad] : Inport  Port=3
  Dynamic Pressure [Pa] : Inport  Port=4
  Angle of Attack [rad] : Inport  Port=5
  Sideslip Angle [rad] : Inport  Port=6
  Airspeed [m/s] : Inport  Port=7
  Add : Sum  Inputs=+++
  Aerodynamic Forces and Moments Coef Axis Variant : Subsystem  Variant=on
  Base Airframe : Subsystem
  Control Derivatives : Subsystem
  Dynamic Derivatives : Subsystem
  Fxyz Mxzy : Outport
  wires:
  Base Airframe/1(C6) -> Add/1
  Dynamic Derivatives/1(dC6) -> Add/2
  Sideslip Angle [rad]/1 -> Base Airframe/2(Sideslip Angle [rad])
  Angle of Attack [rad]/1 -> Base Airframe/1(Angle of Attack [rad]), Control Derivatives/2(Angle of Attack [rad]), Dynamic Derivatives/3(Angle of Attack [rad])
  Body Rotational Rates [rad/s]/1 -> Dynamic Derivatives/2(Body Rotational Rate [rad/s])
  Airspeed [m/s]/1 -> Dynamic Derivatives/1(Airspeed [m/s])
  Surface Positions [rad]/1 -> Control Derivatives/1(Surface Positions [rad])
  Control Derivatives/1(dC6) -> Add/3
  Add/1 -> Aerodynamic Forces and Moments Coef Axis Variant/1(Coef)
  Body Velocity [m/s]/1 -> Aerodynamic Forces and Moments Coef Axis Variant/3(Body Velocity [m/s])
  Dynamic Pressure [Pa]/1 -> Aerodynamic Forces and Moments Coef Axis Variant/2(Dynamic Pressure [Pa])
  Aerodynamic Forces and Moments Coef Axis Variant/1(Fxyz Mxyz) -> Fxyz Mxzy/1

== system uas_sim/Vehicle/Forces and Moments/Gravitational ==
  Gravity [m/s/s] : Inport
  DCM_be : Inport  Port=2
  Gravity Moment : Constant  Value=[0 0 0]
  Mux : Mux  Inputs=2
  Product : Product
  Product1 : Product  Multiplication=Matrix(*)
  Reshape : Reshape  OutputDimensionality=Column vector (2-D)
  Reshape1 : Reshape
  UAV Mass : Constant  Value=Aircraft.Mass.mass_kg
  Fxyz Mxyz : Outport
  wires:
  UAV Mass/1 -> Product/2
  Product/1 -> Product1/2  "Gravity Force NED [N]"
  DCM_be/1 -> Product1/1
  Gravity Moment/1 -> Mux/2
  Mux/1 -> Fxyz Mxyz/1
  Reshape/1 -> Product/1
  Gravity [m/s/s]/1 -> Reshape/1
  Reshape1/1 -> Mux/1
  Product1/1 -> Reshape1/1  "Gravity Force Body [N]"

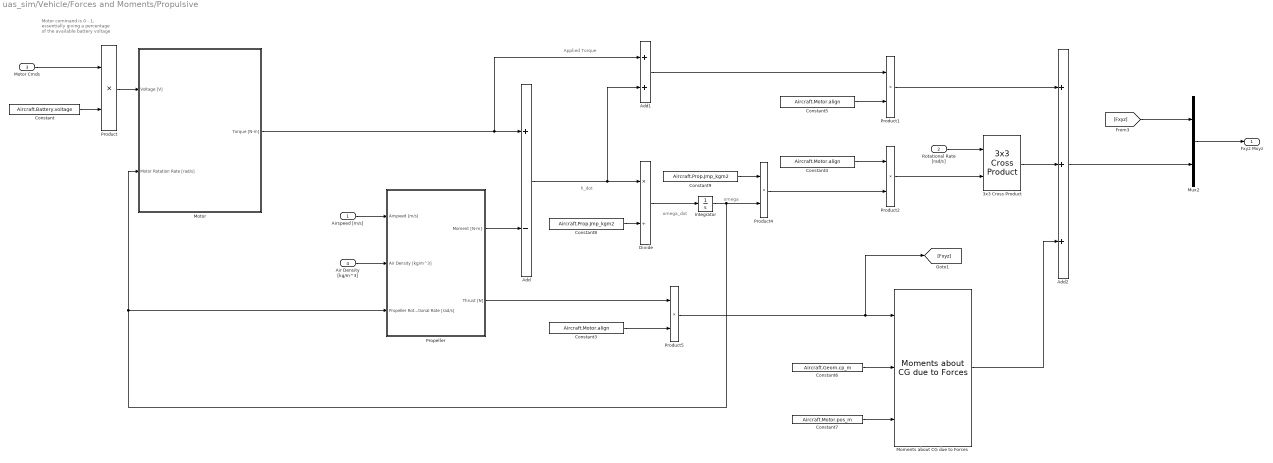
== system uas_sim/Vehicle/Forces and Moments/Propulsive ==
  note: Applied Torque
  note: omega_dot
  note: Motor command is 0 - 1,
      | essentially giving a percentage
      | of the available battery voltage
  note: h_dot
  note: omega
  Airspeed [m/s] : Inport
  Rotational Rate [rad/s] : Inport  Port=2
  Motor Cmds : Inport  Port=3
  Air Density [kg/m^3] : Inport  Port=4
  3x3 Cross Product : sharedutil/3x3 Cross Product  aMode=aMode
  Add : Sum  Inputs=+-
  Add1 : Sum
  Add2 : Sum  Inputs=+++
  Constant : Constant  Value=Aircraft.Battery.voltage
  Constant3 : Constant  Value=Aircraft.Motor.align
  Constant4 : Constant  Value=Aircraft.Motor.align
  Constant5 : Constant  Value=Aircraft.Motor.align
  Constant6 : Constant  Value=Aircraft.Geom.cp_m
  Constant7 : Constant  Value=Aircraft.Motor.pos_m
  Constant8 : Constant  Value=Aircraft.Prop.Jmp_kgm2
  Constant9 : Constant  Value=Aircraft.Prop.Jmp_kgm2
  Divide : Product  Inputs=*/
  Integrator : Integrator  InitialCondition=InitCond.engine_speed_radps  LowerSaturationLimit=1
  Moments about CG due to Forces : aerolibbdyn/Moments about CG  due to Forces
  Motor : Subsystem
  Mux2 : Mux  Inputs=2
  Product{,1..2,4..5} (5 alike) : Product
  Propeller : Subsystem
  Fxyz Mxyz : Outport
  wires:
  Integrator/1 -> Product4/2, Propeller/3(Propeller Rotational Rate [rad/s]), Motor/2(Motor Rotation Rate [rad/s])
  [Fxyz] -> Mux2/1
  Constant4/1 -> Product2/1
  Motor/1(Torque [N-m]) -> Add1/1, Add/1
  Add1/1 -> Product1/1
  Product/1 -> Motor/1(Voltage [V])
  Moments about CG due to Forces/1 -> Add2/3
  Product1/1 -> Add2/1
  Add2/1 -> Mux2/2
  Constant9/1 -> Product4/1
  Propeller/2(Thrust [N]) -> Product5/1
  3x3 Cross Product/1 -> Add2/2
  Mux2/1 -> Fxyz Mxyz/1
  Constant/1 -> Product/2
  Product5/1 -> [Fxyz], Moments about CG due to Forces/1
  Constant3/1 -> Product5/2
  Divide/1 -> Integrator/1
  Add/1 -> Add1/2, Divide/1
  Propeller/1("Moment [N-m}") -> Add/2
  Constant6/1 -> Moments about CG due to Forces/2
  Rotational Rate [rad/s]/1 -> 3x3 Cross Product/1
  Air Density [kg/m^3]/1 -> Propeller/2(Air Density [kg/m^3])
  Product4/1 -> Product2/2
  Constant7/1 -> Moments about CG due to Forces/3
  Constant8/1 -> Divide/2
  Product2/1 -> 3x3 Cross Product/2
  Constant5/1 -> Product1/2
  Motor Cmds/1 -> Product/1
  Airspeed [m/s]/1 -> Propeller/1(Airspeed [m/s])

== system uas_sim/Vehicle/Vehicle Model/Norm ==
  2D Vector : Inport
  Product : Product
  Sqrt : Sqrt
  Sum of Elements : Sum  Inputs=+
  Norm : Outport
  wires:
  2D Vector/1 -> Product/2, Product/1
  Product/1 -> Sum of Elements/1
  Sum of Elements/1 -> Sqrt/1
  Sqrt/1 -> Norm/1
